simulink model "P2_Q6"  (Simulink 9.2)
settings: Solver=VariableStepAuto  StartTime=0.0  StopTime=10.0  RelTol=1e-3
undefined symbols (not defined in the file or in its folder): x1_nod, x2_nod
settings Model: Creator=vassili  LastModifiedBy=vassili
settings DataIOCC: LimitDataPoints=off  SaveFormat=Dataset  SignalLoggingSaveFormat=Dataset
settings OptimizationCC: LifeSpan=auto
settings DebuggingCC: UnderspecifiedInitializationDetection=Simplified  MergeDetectMultiDrivingBlocksExec=error  FcnCallInpInsideContextMsg=error  StateNameClashWarn=none  LibraryContextMissingDiagnostic=none  SFUnexpectedBacktrackingDiag=error  SFNoUnconditionalDefaultTransitionDiag=error  SFExecutionAtInitializationDiag=warning
settings HardwareCC: ProdBitPerPointer=64  ProdBitPerSizeT=64  ProdBitPerPtrDiffT=64  ProdLargestAtomicFloat=Float  ProdIntDivRoundTo=Zero  ProdEndianess=LittleEndian  ProdWordSize=64  ProdHWDeviceType=Intel->x86-64 (Windows64)
settings ModelReferenceCC: PropagateSignalLabelsOutOfModel=on
settings CodeAppCC: StateflowObjectComments=off
settings GRTTargetCC: TargetLangStandard=C99 (ISO)  GeneratePreprocessorConditionals=Use local settings  CombineOutputUpdateFcns=on  GRTInterface=off
settings ConfigComp: CovMetricSettings=dwe  CovHtmlReporting=off  CovSaveCumulativeToWorkspaceVar=off  CovSaveSingleToWorkspaceVar=off  CovExternalEMLEnable=on

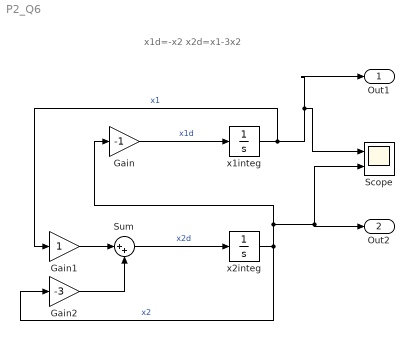
== system P2_Q6 ==
  note: x1d=-x2
      | x2d=x1-3x2
  Gain : Gain  Gain=-1
  Gain1 : Gain
  Gain2 : Gain  Gain=-3
  Scope : Scope  NumInputPorts=2
  Sum : Sum  Inputs=|++
  x1integ : Integrator  InitialCondition=x1_nod
  x2integ : Integrator  InitialCondition=x2_nod
  Out1 : Outport
  Out2 : Outport  Port=2
  wires:
  x1integ/1 -> Gain1/1, Scope/1, Out1/1  "x1"
  x2integ/1 -> Gain2/1, Scope/2, Out2/1, Gain/1  "x2"
  Gain/1 -> x1integ/1  "x1d"
  Sum/1 -> x2integ/1  "x2d"
  Gain1/1 -> Sum/1
  Gain2/1 -> Sum/2
